simulink model "FourQuadrantChopper"  (R2024b)
settings: Solver=FixedStepAuto  StartTime=0.0  StopTime=inf  FixedStep=10e-6  RelTol=1e-3
libraries: spsMosfetLib x4, spsDCVoltageSourceLib x2, spsCurrentMeasurementLib x1, simulink x1, spsSeriesRLCBranchLib x1, spsVoltageMeasurementLib x1, sps_lib x1
settings Model: Creator=Ketan  LastModifiedBy=Ketan

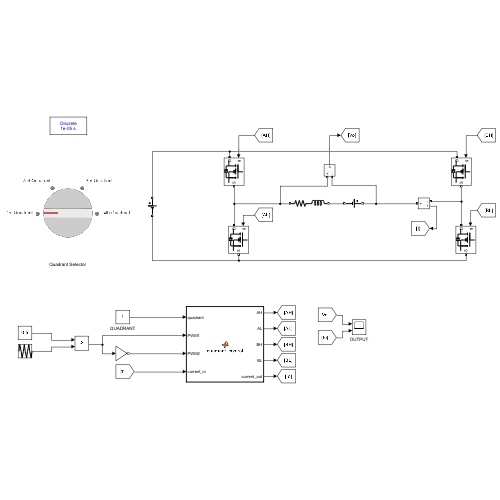
[thumbnail: Simulink's stored preview of the top-level diagram]
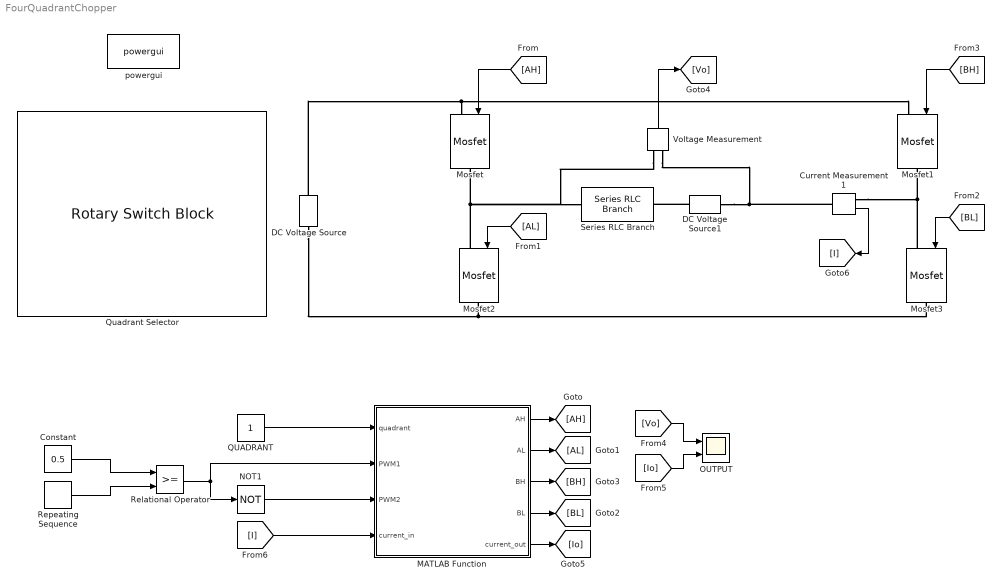
== system FourQuadrantChopper ==
  Constant : Constant  Value=0.5
  Current Measurement1 : spsCurrentMeasurementLib/Current Measurement  PhasorSimulation=off  OutputType=Complex  PSBequivalent=0
  DC Voltage Source : spsDCVoltageSourceLib/DC Voltage Source  Amplitude=100  Measurements=None
  DC Voltage Source1 : spsDCVoltageSourceLib/DC Voltage Source  Amplitude=100  Measurements=None
  MATLAB Function : MATLAB Function  TreatAsAtomicUnit=on
  Mosfet{,1..3} (4 alike) : spsMosfetLib/Mosfet  Ron=0.1  Lon=0  Rd=0.01  Vfd=0  IC=0  Rs=1e5  Cs=inf  Measurements=off
  NOT1 : Logic  Operator=NOT  IconShape=distinctive  AllPortsSameDT=off  OutDataTypeStr=boolean
  OUTPUT : Scope  NumInputPorts=2
  QUADRANT : Constant
  Quadrant Selector : RotarySwitchBlock  LabelPosition=Hide
      settings: Values={{'1st Quadrant', '2nd Quadrant', '3rd Quadrant', '4th Quadrant'}, [1 2 3 4]}
  Relational Operator : RelationalOperator  OutDataTypeStr=boolean  RndMeth=Simplest  InputSameDT=off
  Repeating Sequence : simulink/Sources/Repeating Sequence  rep_seq_t=[0 0.25 0.5 0.75 1]  rep_seq_y=[0 1 0 -1 0]
  Series RLC Branch : spsSeriesRLCBranchLib/Series RLC Branch  LConnTagsString=__new0  RConnTagsString=__new0  BranchType=RL  Resistance=3  Inductance=0.2  SetiL0=off  InitialCurrent=0  Capacitance=1e-6  Setx0=off  InitialVoltage=0  Measurements=None
  Voltage Measurement : spsVoltageMeasurementLib/Voltage Measurement  PhasorSimulation=off  OutputType=Complex  PSBequivalent=0
  powergui : sps_lib/powergui  Priority=1  SimulationMode=Discrete  SampleTime=10e-6  frequency=60  Iterations=50  frequencyindice=0  Pbase=100e6  ErrMax=1e-4  UnitsV=kV  UnitsW=MW  buscounter=0  FunctionMessages=off  echomessages=off  EnableUseOfTLC=off  CurrentSourceSwitches=off  DisableSnubberDevices=off  DisableRonSwitches=off  DisableVfSwitches=off  DisplayEquations=off  AutomaticDiscreteSolvers=off  SolverType=Tustin/Backward Euler (TBE)  Interpol=off  ExternalGateDelay=off  methode=off  Ts=100  x0status=blocks  SPID=on  SwTol=0  HookPort=off  NonlinearTolerance=1e-4  nMaxIteration=100  ContinueOnMaxIteration=off  RestoreLinks=warning  ResistiveCurrentMeasurement=off  Frange=[0:2:500]  Ylog=off  Xlog=on  ShowGrid=off  save=off  variable=ZData  structure=0  ZoomFFT=off  StartTime=0.0  cycles=1  DisplayStyle=1  fundamental=60  FreqAxis=off  MaxFrequency=1000  frequencyindicesteady=1  RmsSteady=1  display=off
  wires:
  Constant/1 -> Relational Operator/1
  Repeating Sequence/1 -> Relational Operator/2
  Relational Operator/1 -> MATLAB Function/2(PWM1), NOT1/1
  NOT1/1 -> MATLAB Function/3(PWM2)
  QUADRANT/1 -> MATLAB Function/1(quadrant)
  MATLAB Function/1(AH) -> [AH]
  [AH] -> Mosfet/1
  MATLAB Function/2(AL) -> [AL]
  [AL] -> Mosfet2/1
  MATLAB Function/4(BL) -> [BL]
  [BL] -> Mosfet3/1
  MATLAB Function/3(BH) -> [BH]
  [BH] -> Mosfet1/1
  Voltage Measurement/1 -> [Vo]
  [Vo] -> OUTPUT/1
  MATLAB Function/5(current_out) -> [Io]
  [Io] -> OUTPUT/2
  Current Measurement1/1 -> [I]
  [I] -> MATLAB Function/4(current_in)
  connections:
  DC Voltage Source/RConn1 -- Mosfet/LConn1 -- Mosfet1/LConn1
  DC Voltage Source/LConn1 -- Mosfet2/RConn1 -- Mosfet3/RConn1
  Mosfet3/LConn1 -- Current Measurement1/RConn1 -- Mosfet1/RConn1
  DC Voltage Source1/LConn1 -- Series RLC Branch/RConn1
  Voltage Measurement/LConn2 -- DC Voltage Source1/RConn1 -- Current Measurement1/LConn1
  Mosfet2/LConn1 -- Series RLC Branch/LConn1 -- Voltage Measurement/LConn1 -- Mosfet/RConn1

== matlab function FourQuadrantChopper/MATLAB Function ==
  data: quadrant input; AH output; PWM1 input; PWM2 input; current_in input; AL output; BH output; BL output; current_out output
function [AH, AL, BH, BL, current_out] = quadrant_control(quadrant, PWM1, PWM2, current_in)
% Inputs:
%   quadrant: 1, 2, 3, or 4 (operation mode)
%   PWM1: Primary PWM signal
%   PWM2: Complementary PWM signal (~PWM1)
%   current_in: Measured current (can be +ve or -ve)
%
% Outputs:
%   AH, AL, BH, BL: Gate signals (logical)
%   current_out: Current with polarity reversed in Q2/Q3

% Initialize all gate signals as OFF (logical false)
AH = false; AL = false; BH = false; BL = false;

% Current polarity handling (reverse in Q2/Q3)
current_out = current_in; % Default
if quadrant == 2 || quadrant == 3
    current_out = -current_in; % Reverse polarity for regeneration modes
end

% Switching logic based on quadrant
switch quadrant
    case 1 % 1st Quadrant (+V, +I): Forward motoring
        AH = logical(PWM1); 
        AL = logical(PWM2); 
        BH = false;         % BH OFF
        BL = true;          % BL always ON 
        
    case 2 % 2nd Quadrant (+V, -I): Forward regeneration
        AH = logical(PWM1);
        AL = logical(PWM2); 
        BH = false;        
        BL = true;          
        
    case 3 % 3rd Quadrant (-V, -I): Reverse motoring
        AH = false;         % AH OFF
        AL = true;          % AL always ON (freewheeling path)
        BH = logical(PWM1);
        BL = logical(PWM2); 
        
    case 4 % 4th Quadrant (-V, +I): Reverse regeneration
        AH = false;         
        AL = true;          
        BH = logical(PWM1); 
        BL = logical(PWM2); 
end
end
